simulink model "DoubleLeafWallOriginal"  (R2021b)
settings: Solver=VariableStepAuto  StartTime=0.0  StopTime=60  RelTol=1e-3
values from neighbouring files (symbols this model uses):
  c = 3    [plotX2vsW.m]    (also in plotX2vsWLowerFreq.m; plotX2vsWaddedCw.m; simulateX2vsWaddedCa.m)
  cw = 500    [plotX2vsWaddedCw.m]    (also in simulateX2vsWaddedCa.m)
  F = 10    [plotX2vsW.m]    (also in plotX2vsWLowerFreq.m; plotX2vsWaddedCw.m; simulateX2vsWaddedCa.m)
  k = 171080    [plotX2vsW.m]    (also in plotX2vsWLowerFreq.m; plotX2vsWaddedCw.m; simulateX2vsWaddedCa.m)
  m1 = 1    [plotX2vsW.m]    (also in plotX2vsWLowerFreq.m; plotX2vsWaddedCw.m; simulateX2vsWaddedCa.m)
  m2 = 1    [plotX2vsW.m]    (also in plotX2vsWLowerFreq.m; plotX2vsWaddedCw.m; simulateX2vsWaddedCa.m)
  w = zeros(815,1)    [plotX2vsW.m]    (also in plotX2vsWLowerFreq.m = zeros(175,1); plotX2vsWaddedCw.m; simulateX2vsWaddedCa.m = 125:5:940)
settings Model: Creator=vsor436  LastModifiedBy=ltan820
settings SolverCC: AlgebraicLoopSolver=TrustRegion
settings DebuggingCC: SFMachineParentedDataDiag=warning

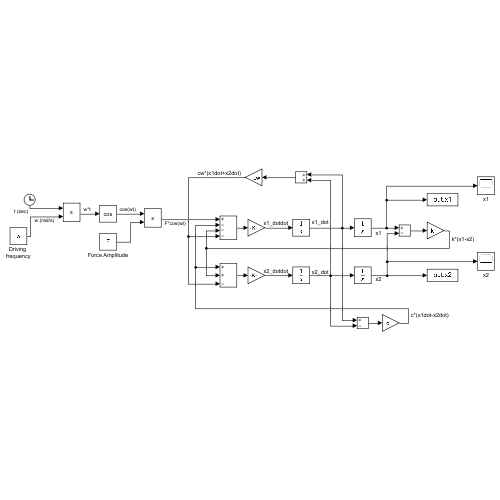
[thumbnail: Simulink's stored preview of the top-level diagram]
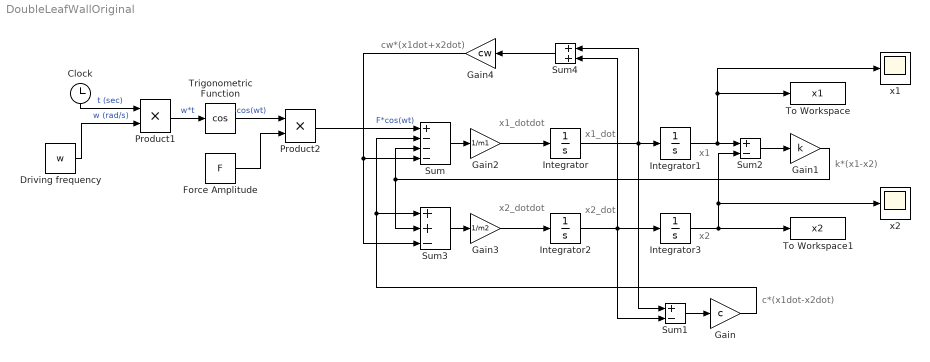
== system DoubleLeafWallOriginal ==
  note: k*(x1-x2)
  note: cw*(x1dot+x2dot)
  note: c*(x1dot-x2dot)
  note: x1_dotdot
  note: x2
  note: x1
  note: x1_dot
  note: x2_dot
  note: x2_dotdot
  Clock : Clock
  Driving frequency : Constant  Value=w
  Force Amplitude : Constant  Value=F
  Gain : Gain  Gain=c
  Gain1 : Gain  Gain=k
  Gain2 : Gain  Gain=1/m1
  Gain3 : Gain  Gain=1/m2
  Gain4 : Gain  Gain=cw
  Integrator : Integrator
  Integrator1 : Integrator  UpperSaturationLimit=0.01  LowerSaturationLimit=-0.01  WrappedStateUpperValue=0.01  WrappedStateLowerValue=-0.01
  Integrator2 : Integrator
  Integrator3 : Integrator
  Product1 : Product
  Product2 : Product
  Sum : Sum  Inputs=+---
  Sum1 : Sum  Inputs=+-
  Sum2 : Sum  Inputs=+-
  Sum3 : Sum  Inputs=++-
  Sum4 : Sum
  To Workspace : ToWorkspace  VariableName=x1  SampleTime=-1
  To Workspace1 : ToWorkspace  VariableName=x2  SampleTime=-1
  Trigonometric Function : Trigonometry  Operator=cos
  x1 : Scope
  x2 : Scope
  wires:
  Product1/1 -> Trigonometric Function/1  "w*t"
  Trigonometric Function/1 -> Product2/1  "cos(wt)"
  Clock/1 -> Product1/1  "t (sec)"
  Driving frequency/1 -> Product1/2  "w (rad/s)"
  Force Amplitude/1 -> Product2/2
  Product2/1 -> Sum/1  "F*cos(wt)"
  Integrator/1 -> Sum1/1, Sum4/1, Integrator1/1
  Sum1/1 -> Gain/1
  Gain/1 -> Sum/2, Sum3/1
  Sum2/1 -> Gain1/1
  Gain1/1 -> Sum/3, Sum3/2
  Sum/1 -> Gain2/1
  Gain2/1 -> Integrator/1
  Gain3/1 -> Integrator2/1
  Sum3/1 -> Gain3/1
  Integrator1/1 -> x1/1, To Workspace/1, Sum2/1
  Integrator3/1 -> Sum2/2, x2/1, To Workspace1/1
  Integrator2/1 -> Sum4/2, Integrator3/1, Sum1/2
  Sum4/1 -> Gain4/1
  Gain4/1 -> Sum3/3, Sum/4
